simulink model "StmStrLogger"  (R2024a)
settings: Solver=VariableStepAuto  StartTime=0.0  StopTime=10.0  RelTol=1e-3
settings Model: Creator=user  LastModifiedBy=user

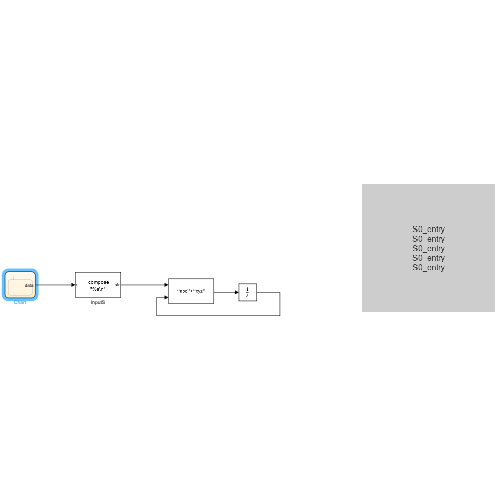
[thumbnail: Simulink's stored preview of the top-level diagram]
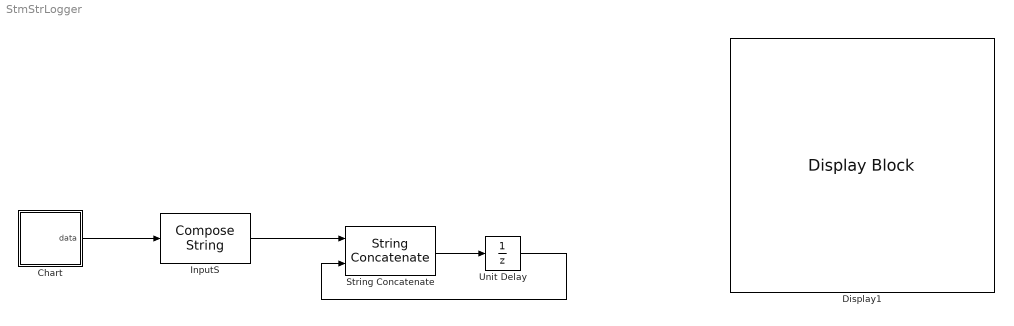
== system StmStrLogger ==
  Chart : Stateflow chart  TreatAsAtomicUnit=on
  Display1 : DisplayBlock  LabelPosition=Hide  Transparency=1
  InputS : ComposeString  Format="\"%s\\n\""
  String Concatenate : StringConcatenate
  Unit Delay : UnitDelay  SampleTime=-1  HasFrameUpgradeWarning=on
  wires:
  String Concatenate/1 -> Unit Delay/1
  InputS/1 -> String Concatenate/1
  Unit Delay/1 -> String Concatenate/2
  Chart/1(data) -> InputS/1

== stateflow chart StmStrLogger/Chart ==
  state S0_
    entry: data="S0_entry";
  (default) -> S0_
  data: data output
